simulink model "test_trigger_2"  (R2018a)
settings: Solver=VariableStepAuto  StartTime=0.0  StopTime=0.001  RelTol=1e-3
values from neighbouring files (symbols this model uses):
  trigger = true    [final_test.m]    (also in main_file.m; vel_measurement_final.m)
libraries: TcAdsLib x2
settings Model: Creator=bschumann  LastModifiedBy=bschumann

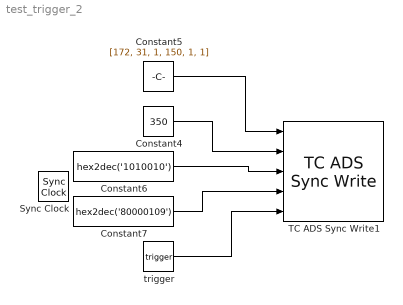
== system test_trigger_2 ==
  Constant4 : Constant  Value=350  OutDataTypeStr=uint16
  Constant5 : Constant  Value=[172, 31, 1, 150, 1, 1]  OutDataTypeStr=uint8
  Constant6 : Constant  Value=hex2dec('1010010')  OutDataTypeStr=uint32
  Constant7 : Constant  Value=hex2dec('80000109')  OutDataTypeStr=uint32
  Sync Clock : TcAdsLib/Utilities/Sync Clock  OutputPortSelect=None  InputPortSelect=None
      settings: SourceProductName=Beckhoff TwinCAT ADS Interface
  TC ADS Sync Write1 : TcAdsLib/Synchronous/TC ADS Sync Write  SampleTime=-1  AbortSimulationOnAdsError=off  WriteDataType=boolean  WriteDataDim=1  WriteDataColToRowMajor=on  AdsTimeout=1  DirectFeedThrough=off  CreateSignalLabels=on  CodeGenConnectType=DataArea (OutputSrc)
      settings: SourceProductName=Beckhoff TwinCAT ADS Interface
  trigger : Constant  Value=trigger  OutDataTypeStr=boolean
  wires:
  trigger/1 -> TC ADS Sync Write1/5
  Constant5/1 -> TC ADS Sync Write1/1
  Constant4/1 -> TC ADS Sync Write1/2
  Constant7/1 -> TC ADS Sync Write1/4
  Constant6/1 -> TC ADS Sync Write1/3
